simulink model "Technical_Test_2_model"  (R2024a)
settings: Solver=VariableStepAuto  StartTime=0.0  StopTime=1800  MaxStep=1  RelTol=1e-3
undefined symbols (not defined in the file): Af, Cd, Cr, DiscIntNeverNeededParam, g, M, rho, Rw, theta
settings Model: Creator=Roshan_PC  LastModifiedBy=Roshan_PC

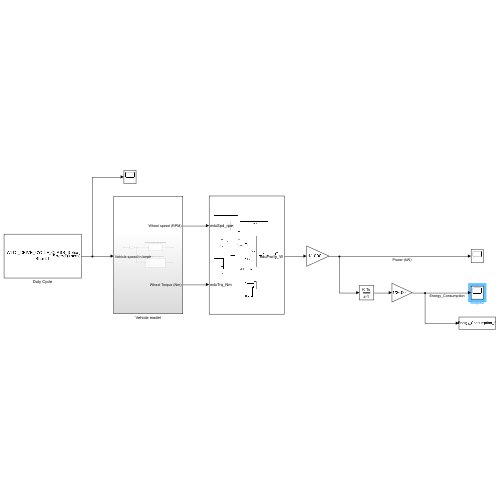
[thumbnail: Simulink's stored preview of the top-level diagram]
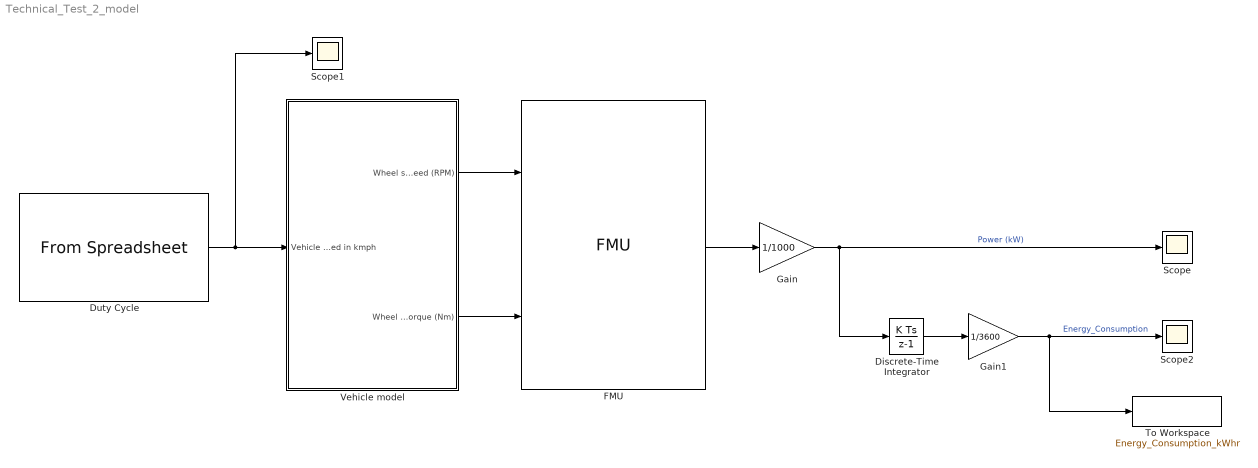
== system Technical_Test_2_model ==
  Discrete-Time Integrator : DiscreteIntegrator  SampleTime=-1  ICPrevOutput=DiscIntNeverNeededParam  ICPrevScaledInput=DiscIntNeverNeededParam
  Duty Cycle : FromSpreadsheet  FileName=WLTC_DRIVE_CYCLE_CLASS_3.xlsx
  FMU : FMU  FMUName=eduModel.fmu  FMUDebugLogging=on  FMUMode=CoSimulation  FMUCreateBusObject=off  FMUInitializeEnumObject=off  FMUCachedDialogLayout="{\"Geometry\":[1315,326,535,467],\"ParameterColumnsWidthConfig\":\"{\\\"columns\\\":[{\\\"name\\\":\\\"Parameter\\\",\\\"width\\\":144},{\\\"name\\\":\\\"Value\\\",\\\"width\\\":115},{\\\"name\\\":\\\"Unit\\\",\\\"width\\\":107},{\\\"name\\\":\\\"Description\\\",\\\"width\\\":149}]}\",\"InputColumnsWidthConfig\":[],\"OutputColumnsWidthConfig\":[]}"  motorConfig=3  ratio=15  mask(eduModel [Co-Simulation, v2.0]){}
      mask Display:
      | if (exist([Simulink.fileGenControl('get','CacheFolder') '\slprj\_fmu\33689cabd0e25a119382c1209330c931\eduModel\model.png'],'file'))
      |     image([Simulink.fileGenControl('get','CacheFolder') '\slprj\_fmu\33689cabd0e25a119382c1209330c931\eduModel\model.png']);
      | else
      |     disp('eduModel');
      | end
      | port_label('output',1,'eduPwrIn_W');
      | port_label('input',1,'eduSpd_rpm');
      | port_label('input',2,'eduTrq_Nm');
  Gain : Gain  Gain=1/1000
  Gain1 : Gain  Gain=1/3600
  Scope : Scope
  Scope1 : Scope
  Scope2 : Scope
  To Workspace : ToWorkspace  VariableName=Energy_Consumption_kWhr  SaveFormat=Timeseries  SampleTime=-1
  Vehicle model : Subsystem
  wires:
  Duty Cycle/1 -> Scope1/1, Vehicle model/1(Vehicle speed in kmph)
  Vehicle model/1(Wheel speed (RPM)) -> FMU/1
  Vehicle model/2(Wheel Torque (Nm)) -> FMU/2
  FMU/1 -> Gain/1
  Gain/1 -> Scope/1, Discrete-Time Integrator/1  "Power (kW)"
  Discrete-Time Integrator/1 -> Gain1/1
  Gain1/1 -> Scope2/1, To Workspace/1  "Energy_Consumption"

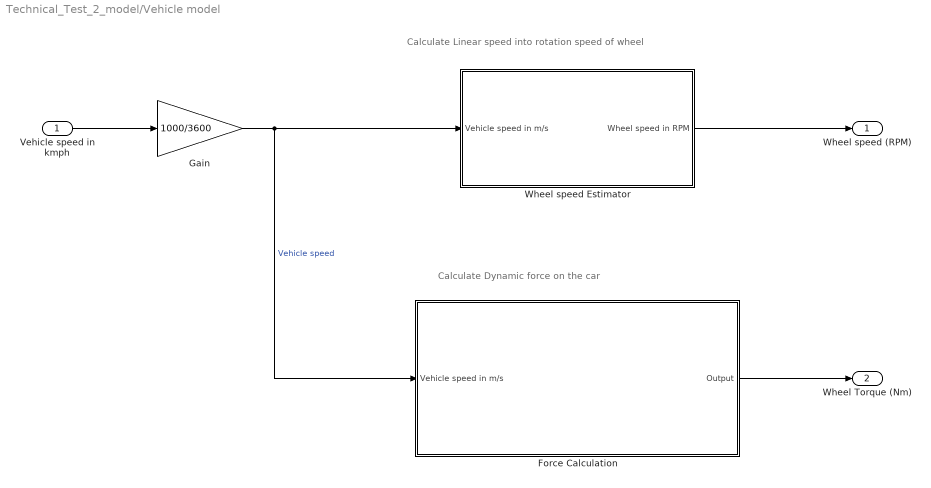
== system Technical_Test_2_model/Vehicle model ==
  note: Calculate Dynamic force on the car
  note: Calculate Linear speed into rotation speed of wheel
  Vehicle speed in kmph : Inport
  Force Calculation : Subsystem
  Gain : Gain  Gain=1000/3600
  Wheel speed Estimator : Subsystem
  Wheel speed (RPM) : Outport
  Wheel Torque (Nm) : Outport  Port=2
  wires:
  Vehicle speed in kmph/1 -> Gain/1
  Gain/1 -> Force Calculation/1(Vehicle speed in m/s), Wheel speed Estimator/1(Vehicle speed in m/s)  "Vehicle speed"
  Force Calculation/1(Output) -> Wheel Torque (Nm)/1
  Wheel speed Estimator/1(Wheel speed in RPM) -> Wheel speed (RPM)/1

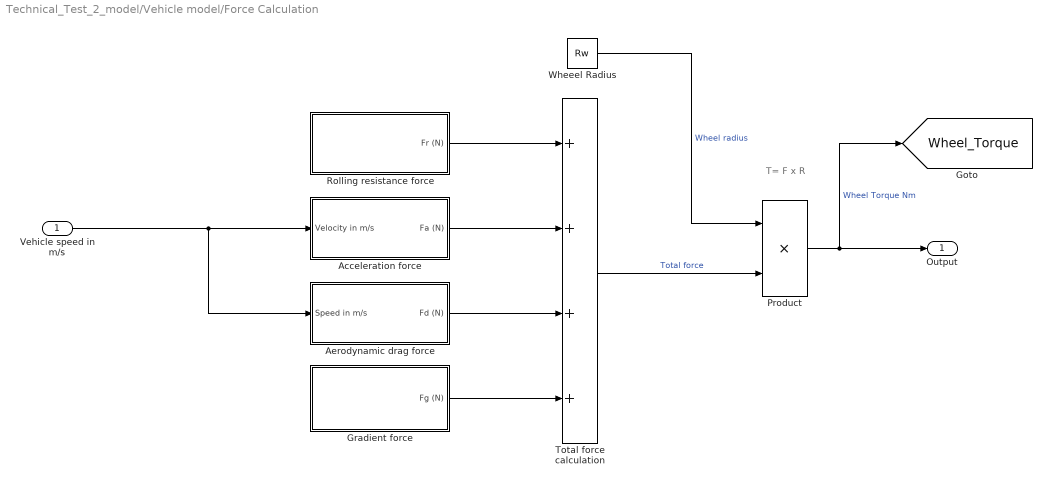
== system Technical_Test_2_model/Vehicle model/Force Calculation ==
  note: T= F x R
  Vehicle speed in m/s : Inport
  Acceleration force : Subsystem
  Aerodynamic drag force : Subsystem
  Gradient force : Subsystem
  Product : Product
  Rolling resistance force : Subsystem
  Total force calculation : Sum  Inputs=++++
  Wheeel Radius : Constant  Value=Rw
  Output : Outport
  tag scope: Wheel_Torque=global
  wires:
  Vehicle speed in m/s/1 -> Aerodynamic drag force/1(Speed in m/s), Acceleration force/1("Velocity in m/s ")
  Rolling resistance force/1(Fr (N)) -> Total force calculation/1
  Acceleration force/1(Fa (N)) -> Total force calculation/2
  Aerodynamic drag force/1(Fd (N)) -> Total force calculation/3
  Gradient force/1(Fg (N)) -> Total force calculation/4
  Wheeel Radius/1 -> Product/1  "Wheel radius"
  Total force calculation/1 -> Product/2  "Total force"
  Product/1 -> [Wheel_Torque], Output/1  "Wheel Torque Nm"

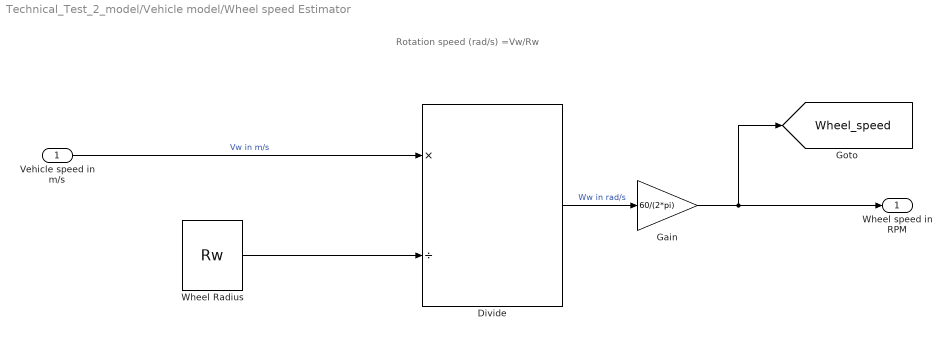
== system Technical_Test_2_model/Vehicle model/Wheel speed Estimator ==
  note: Rotation speed (rad/s) =Vw/Rw
  Vehicle speed in m/s : Inport
  Divide : Product  Inputs=*/
  Gain : Gain  Gain=60/(2*pi)
  Wheel Radius : Constant  Value=Rw
  Wheel speed in RPM : Outport
  tag scope: Wheel_speed=global
  wires:
  Vehicle speed in m/s/1 -> Divide/1  "Vw in m/s"
  Wheel Radius/1 -> Divide/2
  Divide/1 -> Gain/1  "Ww in rad/s"
  Gain/1 -> [Wheel_speed], Wheel speed in RPM/1

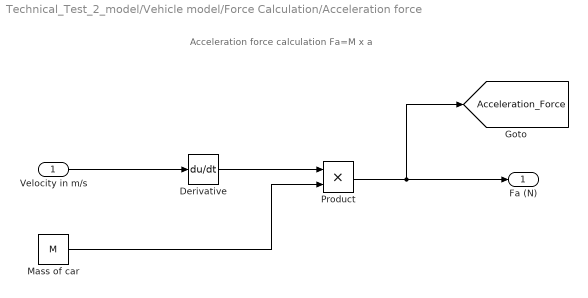
== system Technical_Test_2_model/Vehicle model/Force Calculation/Acceleration force ==
  note: Acceleration force calculation
      | Fa=M x a
  "Velocity in m/s " : Inport
  Derivative : Derivative
  Mass of car : Constant  Value=M
  Product : Product
  Fa (N) : Outport
  tag scope: Acceleration_Force=global
  wires:
  "Velocity in m/s "/1 -> Derivative/1
  Mass of car/1 -> Product/2
  Derivative/1 -> Product/1
  Product/1 -> [Acceleration_Force], Fa (N)/1

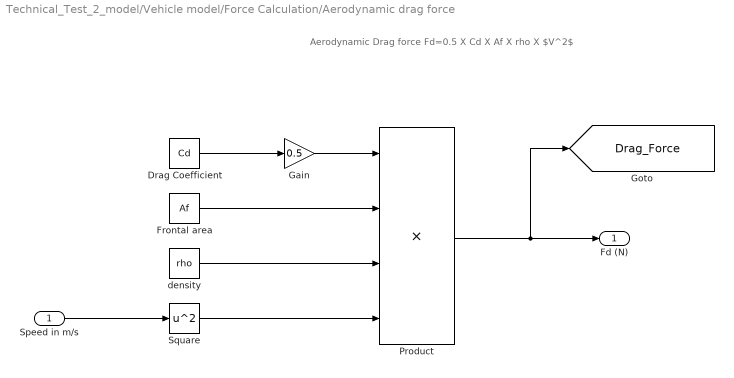
== system Technical_Test_2_model/Vehicle model/Force Calculation/Aerodynamic drag force ==
  note: Aerodynamic Drag force
      | Fd=0.5 X Cd X Af X rho X $V^2$
  Speed in m/s : Inport
  Drag Coefficient : Constant  Value=Cd
  Frontal area : Constant  Value=Af
  Gain : Gain  Gain=0.5
  Product : Product  Inputs=4
  Square : Math  Operator=square
  density : Constant  Value=rho
  Fd (N) : Outport
  tag scope: Drag_Force=global
  wires:
  Speed in m/s/1 -> Square/1
  Drag Coefficient/1 -> Gain/1
  Frontal area/1 -> Product/2
  Gain/1 -> Product/1
  density/1 -> Product/3
  Square/1 -> Product/4
  Product/1 -> [Drag_Force], Fd (N)/1

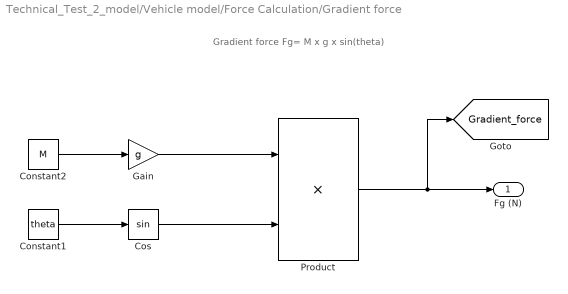
== system Technical_Test_2_model/Vehicle model/Force Calculation/Gradient force ==
  note: Gradient force
      | Fg= M x g x sin(theta)
  Constant1 : Constant  Value=theta
  Constant2 : Constant  Value=M
  Cos : Trigonometry
  Gain : Gain  Gain=g
  Product : Product
  Fg (N) : Outport
  tag scope: Gradient_force=global
  wires:
  Constant2/1 -> Gain/1
  Constant1/1 -> Cos/1
  Product/1 -> [Gradient_force], Fg (N)/1
  Gain/1 -> Product/1
  Cos/1 -> Product/2

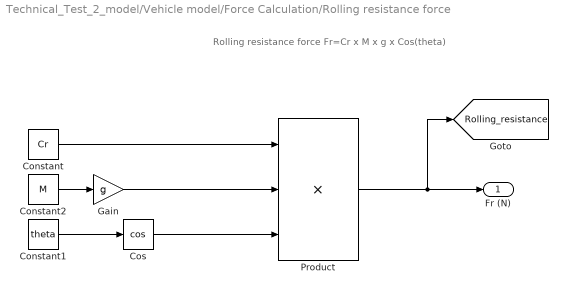
== system Technical_Test_2_model/Vehicle model/Force Calculation/Rolling resistance force ==
  note: Rolling resistance force
      | Fr=Cr x M x g x Cos(theta)
  Constant : Constant  Value=Cr
  Constant1 : Constant  Value=theta
  Constant2 : Constant  Value=M
  Cos : Trigonometry  Operator=cos
  Gain : Gain  Gain=g
  Product : Product  Inputs=3
  Fr (N) : Outport
  tag scope: Rolling_resistance=global
  wires:
  Constant1/1 -> Cos/1
  Constant2/1 -> Gain/1
  Constant/1 -> Product/1
  Gain/1 -> Product/2
  Cos/1 -> Product/3
  Product/1 -> [Rolling_resistance], Fr (N)/1
